simulink model "integral_action"  (R2018b)
settings: Solver=VariableStepAuto  StartTime=0.0  StopTime=50  RelTol=1e-3
values from neighbouring files (symbols this model uses):
  discrete_lqr = c2d(sys, 2*pi/sampling_freq*3, 'zoh')    [integral_augmentation.m]
undefined symbols (not defined in the file or in its folder): DiscIntNeverNeededParam
settings Model: Creator=lorenzoterenzi  LastModifiedBy=lorenzoterenzi

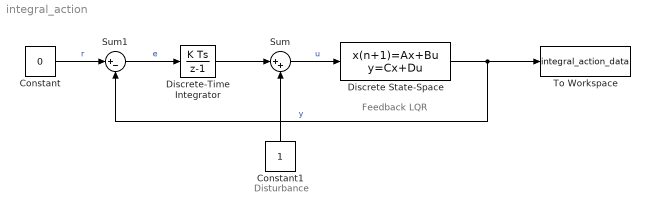
== system integral_action ==
  note: Disturbance
  note: Feedback LQR
  Constant : Constant  Value=0
  Constant1 : Constant
  Discrete State-Space : DiscreteStateSpace  A=discrete_lqr.A  B=discrete_lqr.B  C=discrete_lqr.C  D=discrete_lqr.D  SampleTime=discrete_lqr.Ts
  Discrete-Time Integrator : DiscreteIntegrator  gainval=0.15  SampleTime=-1  ICPrevOutput=DiscIntNeverNeededParam  ICPrevScaledInput=DiscIntNeverNeededParam
  Sum : Sum  Inputs=|++
  Sum1 : Sum  Inputs=|+-
  To Workspace : ToWorkspace  VariableName=integral_action_data  SaveFormat=Timeseries  SampleTime=-1
  wires:
  Discrete State-Space/1 -> To Workspace/1, Sum1/2  "y"
  Sum/1 -> Discrete State-Space/1  "u"
  Constant/1 -> Sum1/1  "r"
  Sum1/1 -> Discrete-Time Integrator/1  "e"
  Discrete-Time Integrator/1 -> Sum/1
  Constant1/1 -> Sum/2
